simulink model "AnalogDiff"  (R2021a)
settings: Solver=FixedStepAuto  StartTime=0.0  StopTime=20  FixedStep=Ts  RelTol=1e-3
values from neighbouring files (symbols this model uses):
  T1 = 5*Ts    (= 0.025)    [differentiator.m]
  T2 = 10*Ts    (= 0.05)    [differentiator.m]
  Ts = 1/fs    (= 0.005)    [differentiator.m]
libraries: simulink x1, pid_lib x1
settings Model: Creator=xiaocy  LastModifiedBy=xiaocy

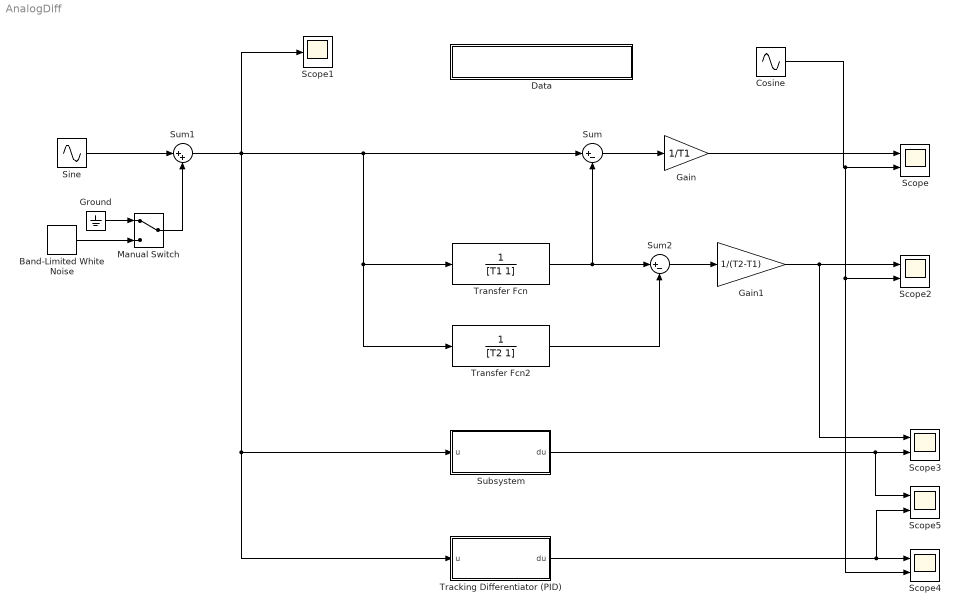
== system AnalogDiff ==
  Band-Limited White Noise : simulink/Sources/Band-Limited White Noise  Cov=0.1^2*Ts  Ts=Ts  seed=[23341]
  Cosine : Sin  Phase=pi/2  SampleTime=0
  Data : Subsystem
      settings: OpenFcn=|
      | Ts = 1e-3;
      | T1 = 10*Ts;
      | T2 = 20*Ts;
      | 
      | sim('AnalogDiff')
      mask Display: disp('Double click to run.')
  Gain : Gain  Gain=1/T1
  Gain1 : Gain  Gain=1/(T2-T1)
  Ground : Ground
  Manual Switch : ManualSwitch
  Scope{,2..5} (5 alike) : Scope  NumInputPorts=2
  Scope1 : Scope
  Sine : Sin  SampleTime=0
  Subsystem : Subsystem
  Sum : Sum  Inputs=|+-
  Sum1 : Sum  Inputs=|++
  Sum2 : Sum  Inputs=|+-
  Tracking Differentiator (PID) : Subsystem
  Transfer Fcn : TransferFcn  Denominator=[T1 1]
  Transfer Fcn2 : TransferFcn  Denominator=[T2 1]
  wires:
  Sum1/1 -> Tracking Differentiator (PID)/1(u), Subsystem/1(u), Sum/1, Transfer Fcn2/1, Transfer Fcn/1, Scope1/1
  Transfer Fcn/1 -> Sum/2, Sum2/1
  Sum/1 -> Gain/1
  Sine/1 -> Sum1/1
  Manual Switch/1 -> Sum1/2
  Band-Limited White Noise/1 -> Manual Switch/2
  Ground/1 -> Manual Switch/1
  Transfer Fcn2/1 -> Sum2/2
  Sum2/1 -> Gain1/1
  Gain/1 -> Scope/1
  Cosine/1 -> Scope2/2, Scope4/2, Scope/2
  Gain1/1 -> Scope3/1, Scope2/1
  Subsystem/1(du) -> Scope5/1, Scope3/2
  Tracking Differentiator (PID)/1(du) -> Scope5/2, Scope4/1

== system AnalogDiff/Data ==

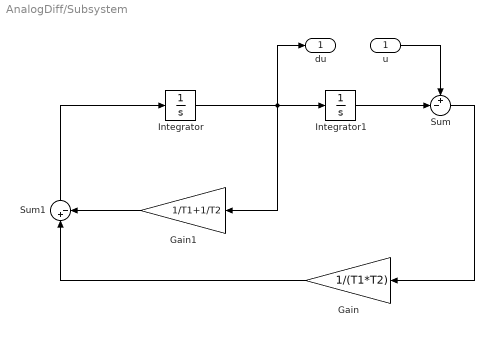
== system AnalogDiff/Subsystem ==
  u : Inport
  Gain : Gain  Gain=1/(T1*T2)
  Gain1 : Gain  Gain=1/T1+1/T2
  Integrator : Integrator
  Integrator1 : Integrator
  Sum : Sum  Inputs=+-|
  Sum1 : Sum  Inputs=|+-
  du : Outport
  wires:
  Integrator/1 -> du/1, Gain1/1, Integrator1/1
  Integrator1/1 -> Sum/2
  u/1 -> Sum/1
  Sum/1 -> Gain/1
  Gain1/1 -> Sum1/2
  Gain/1 -> Sum1/1
  Sum1/1 -> Integrator/1

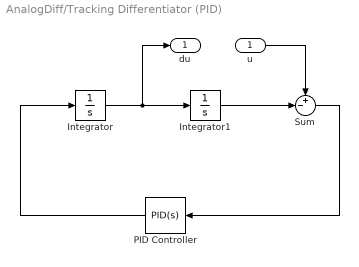
== system AnalogDiff/Tracking Differentiator (PID) ==
  u : Inport
  Integrator : Integrator
  Integrator1 : Integrator
  PID Controller : pid_lib/PID Controller  Controller=PID  Form=Parallel  TimeDomain=Continuous-time  UseExternalTs=off  SampleTime=-1  IntegratorMethod=Forward Euler  FilterMethod=Forward Euler  ControllerParametersSource=internal  P=14.0852125265427  I=5.74309995725058  D=8.48249714466313  UseFilter=on  N=47.5020951212581  TunerSelectOption=Transfer Function Based (PID Tuner App)  InitialConditionSource=internal  InitialConditionForIntegrator=0  InitialConditionForFilter=0  DifferentiatorICPrevScaledInput=0  ExternalReset=none  TrackingMode=off  Kt=1  LimitOutput=off  SatLimitsSource=internal  UpperSaturationLimit=inf  LowerSaturationLimit=-inf  LinearizeAsGain=on  AntiWindupMode=none  Kb=1  POutMin=[]  POutMax=[]  IOutMin=[]  IOutMax=[]  DOutMin=[]  DOutMax=[]  NOutMin=[]  NOutMax=[]  SumOutMin=[]  SumOutMax=[]  SaturationOutMin=[]  SaturationOutMax=[]  PParamMin=[]  PParamMax=[]  IParamMin=[]  IParamMax=[]  DParamMin=[]  DParamMax=[]  NParamMin=[]  NParamMax=[]  KbParamMin=[]  KbParamMax=[]  KtParamMin=[]  KtParamMax=[]  KbOutMin=[]  KbOutMax=[]  KtOutMin=[]  KtOutMax=[]  IntegratorOutMin=[]  IntegratorOutMax=[]  FilterOutMin=[]  FilterOutMax=[]  SumI1OutMin=[]  SumI1OutMax=[]  SumI2OutMin=[]  SumI2OutMax=[]  SumI3OutMin=[]  SumI3OutMax=[]  SumI4OutMin=[]  SumI4OutMax=[]  SumDOutMin=[]  SumDOutMax=[]  DifferentiatorOutMin=[]  DifferentiatorOutMax=[]  FilterDiffOutCoefMin=[]  FilterDiffOutCoefMax=[]  ReciprocalOutMin=[]  ReciprocalOutMax=[]  SumDenOutMin=[]  SumDenOutMax=[]  SumNumOutMin=[]  SumNumOutMax=[]  DivideOutMin=[]  DivideOutMax=[]  UdiffTsProdOutMin=[]  UdiffTsProdOutMax=[]  NTsProdOutMin=[]  NTsProdOutMax=[]  UintegralTsProdOutMin=[]  UintegralTsProdOutMax=[]  UngainTsProdOutMin=[]  UngainTsProdOutMax=[]  IntegratorContinuousStateAttributes=''  IntegratorStateMustResolveToSignalObject=off  IntegratorRTWStateStorageClass=Auto  FilterContinuousStateAttributes=''  FilterStateMustResolveToSignalObject=off  FilterRTWStateStorageClass=Auto  ParallelPVariant=InternalParameters  IdealPVariant=Disabled  IVariant=InternalParameters  DVariant=InternalParameters  IntegratorVariant=Continuous  SatVariant=Disabled  AWVariant=Passthrough  PCopyVariant=Disabled  TRVariant=Disabled  FdbkBlocksVariant=Forward  IdealPFdbkVariant=Disabled  SatFdbkVariant=Disabled  DerivativeFilterVariant=ContFilter  NVariant=InternalParameters  NCopyVariant=Disabled  FilterICVariant=InternalICsFilter  IntegratorICVariant=InternalICs  ExternalResetVariant=Disabled  TRSumVariant=Passthrough  SumFdbkVariant=Disabled  SumVariant=Sum_PID  TsampFilterVariant=InternalTs  TsampNgainVariant=Passthrough  TsampIntegralVariant=Passthrough  ExternalSaturationOutDataTypeStr=Inherit: Same as second input
  Sum : Sum  Inputs=+-|
  du : Outport
  wires:
  PID Controller/1 -> Integrator/1
  Sum/1 -> PID Controller/1
  u/1 -> Sum/1
  Integrator1/1 -> Sum/2
  Integrator/1 -> Integrator1/1, du/1
